simulink model "LinearStateSpaceModelLQR"  (R2014b)
settings: Solver=ode45  StartTime=0.0  StopTime=60  RelTol=1e-6
undefined symbols (not defined in the file): linearized_state_space_model, lqr_gain
settings Model: Creator=NagyZe  LastModifiedBy=NagyZe

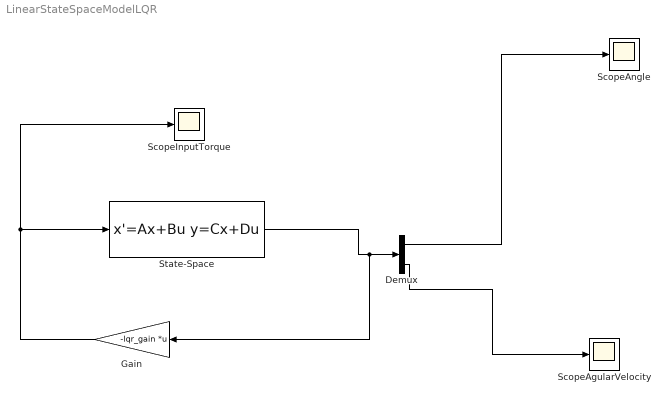
== system LinearStateSpaceModelLQR ==
  Demux : Demux  Outputs=2
  Gain : Gain  Gain=-lqr_gain  Multiplication=Matrix(K*u) (u vector)
  ScopeAgularVelocity : Scope
      settings: TimeRange=10  YMin=-40  YMax=30  SaveName=jointVelocity
  ScopeAngle : Scope
      settings: TimeRange=10  YMin=-0.005  YMax=0.03  SaveName=jointAngle
  ScopeInputTorque : Scope
      settings: YMin=-1  YMax=1  SaveName=torque
  State-Space : StateSpace  A=linearized_state_space_model.A  B=linearized_state_space_model.B  C=eye(4)  D=zeros(4,2)  X0=[0.2 0.1 0 0]
  wires:
  State-Space/1 -> Gain/1, Demux/1
  Demux/2 -> ScopeAgularVelocity/1
  Gain/1 -> ScopeInputTorque/1, State-Space/1
  Demux/1 -> ScopeAngle/1
